simulink model "pump_original_discrete_filter"  (R2018a)
settings: Solver=VariableStepDiscrete  StartTime=0.0  StopTime=40  RelTol=1e-3
values from neighbouring files (symbols this model uses):
  Pl = 22    [pump_ori_perf.mat]
  Ts = 0.0001    [pump_ori_perf.mat]
undefined symbols (not defined in the file or in its folder): DiscIntNeverNeededParam
libraries: fl_lib x13, powerlib x7, powerlib_meascontrol x7, nesl_utility x6, sh_lib x4, simulink x3, dspstat3 x2
settings Model: SimulationMode=accelerator  Creator=siwak  LastModifiedBy=siwak
settings DataIOCC: ReturnWorkspaceOutputs=on
settings OptimizationCC: EfficientMapNaN2IntZero=off
settings DebuggingCC: ReadBeforeWriteMsg=DisableAll  WriteAfterWriteMsg=DisableAll  WriteAfterReadMsg=DisableAll  MultiTaskDSMMsg=none
settings HardwareCC: TargetBitPerPointer=64  TargetBitPerSizeT=64  TargetBitPerPtrDiffT=64  TargetLongLongMode=on  TargetIntDivRoundTo=Zero  TargetEndianess=LittleEndian  TargetWordSize=64  TargetHWDeviceType=MATLAB Host  ProdEqTarget=off
settings CodeAppCC: MaxIdLength=128
settings GRTTargetCC: TargetLangStandard=C89/C90 (ANSI)  CombineOutputUpdateFcns=off  GRTInterface=on

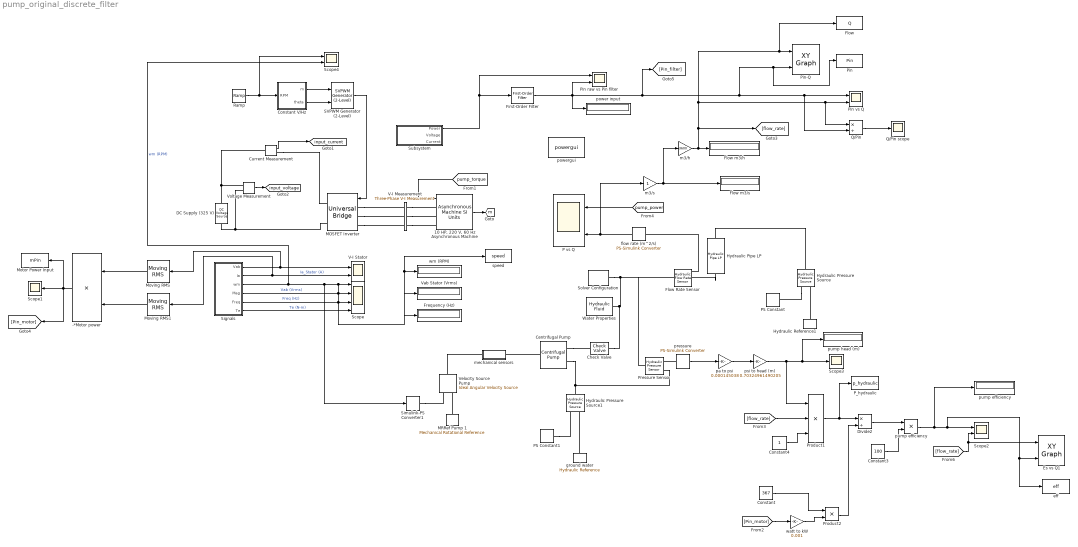
== system pump_original_discrete_filter ==
  " Flow Rate Sensor" : fl_lib/Hydraulic/Hydraulic Sensors/Hydraulic Flow Rate Sensor
      settings: SourceProductName=Simscape
  -*Motor power : Product
  "10 HP, 220 V, 60 Hz Asynchronous Machine" : powerlib/Machines/Asynchronous Machine SI Units  RotorType=Squirrel-cage  PresetModel=No  MechanicalLoad=Torque Tm  ShowDetailedParameters=on  ReferenceFrame=Stationary  Units=SI  MeasurementBus=off  NominalParameters=[ 10*746, 220, 60 ]  Stator="[ 0.435  2*2.0e-3 ]"  Rotor="[ 0.816  2.0e-3 ]"  Cage1=[ 0.022 0.226/377]  Cage2=[ 0.022 0.226/377]  Lm=69.31e-3  Mechanical="[ 0.089  0  2 ]"  PolePairs=2  InitialConditions=[1 90 0 0 0 0 0 0]  SimulateSaturation=off  Saturation=[0 0;0 0]  LoadFlowParameters=2000  TsPowergui=0  TsBlock=-1  IterativeModel=Trapezoidal non iterative  IterativeDiscreteModel=Trapezoidal non iterative  Pmec=0
  Centrifugal Pump : sh_lib/Pumps and Motors/Centrifugal Pump  mdl_type=2  c_1=326.8 Pa/(kg/m^3)  c_2=3.104e+4 Pa*s/kg  c_3=1.097e+7 Pa*s^2/(kg*m^3)  c_4=2.136e+5 Pa*s^2/(kg*m^3)  c_f=0.8  design_del=130 lpm  ref_velocity=1.70e+3 rpm  ref_density=940 kg/m^3  leak_resistance=1e+8 Pa/(m^3/s)  T_const=0.1 N*m  trq_press_coeff=1e-6 N*m/Pa  pump_del_1D="[0    0.0013    0.0041    0.0059    0.0069    0.0082] m^3/s"  press_diff_1D=[50.97 47.08 39.12 31.39 23.6 15.69] psi  pump_del_power_1D="[0    0.0013    0.0041    0.0059    0.0069    0.0082] m^3/s"  power_1D="[0    0.7800    2.1000    2.4000    2.1600    1.7000] HP"  pump_vel_2D=[ 3.2e+3 3.3e+3 3.4e+3 3.5e+3 ] rpm  pump_del_2D=[ 0 50 100 150 200 250 300 350 ] lpm  press_diff_2D=[ 8.3 8.8 9.3 9.9; 7.8 8.3 8.8 9.4; 7.2 7.6 8.2 8.7; 6.5 7 7.5 8; 5.6 6.1 6.6 7.1; 4.7 5.2 5.7 6.2; 3.4 4 4.4 4.9; 2.3 2.7 3.4 3.6 ] bar  pump_del_power_2D=[ 0 50 100 150 200 250 300 350 ] lpm  power_2D=[ 1.223e+3 1.341e+3 1.467e+3 1.6e+3; 1.414e+3 1.551e+3 1.696e+3 1.85e+3; 1.636e+3 1.794e+3 1.962e+3 2.14e+3; 1.941e+3 2.129e+3 2.326e+3 2.54e+3; 2.224e+3 2.439e+3 2.66e+3 2.91e+3; 2.453e+3 2.691e+3 2.947e+3 3.21e+3; 2.757e+3 3.024e+3 3.307e+3 3.608e+3; 2.945e+3 3.23e+3 3.533e+3 3.854e+3 ] W  omega_threshold=1e-9 rad/s  interp_method=1  extrap_method=1
      settings: SourceProductName=Simscape Fluids  SourceProductBaseCode=SH
  "Check Valve " : sh_lib/Valves/Directional Valves/Check Valve  area_max=50670.74790975 mm^2  pres_crack=0.01 psi  pres_max=0.1 psi  C_d=0.7  A_leak=1e-9 m^2  lam_spec=1  B_lam=0.999  Re_cr=12  dynamic=0  tau=0.1 s  area_init=1e-12 m^2
      settings: SourceProductName=Simscape Fluids  SourceProductBaseCode=SH
  Constant : Constant  Value=367
  Constant V/Hz : Subsystem
  Constant3 : Constant  Value=100
  Constant4 : Constant
  Current Measurement : powerlib/Measurements/Current Measurement  PhasorSimulation=off  OutputType=Magnitude  PSBequivalent=0
  DC Supply (325 V) : powerlib/Electrical Sources/DC Voltage Source  Amplitude=325  Measurements=None
  Divide2 : Product  Inputs=*/
  Es vs Q1 : simulink/Sinks/XY Graph  xmin=0  xmax=25  ymin=0  ymax=100  st=-1
  First-Order Filter : powerlib_meascontrol/Filters/First-Order Filter  FilterType=Lowpass  Tc=0.1551  Ts=Ts  Initialize=off  Vac_Init=[0, 0, 60]  Vdc_Init=0  PlotResponse=off  FreqRange="[0,  200,  1]"
      settings: SourceProductName=Simscape Power Systems
  Flow : ToWorkspace  VariableName=Q  SampleTime=-1
      settings: Save2DSignal=2-D array (concatenate along first dimension)
  Flow m3/h : Display
      settings: Decimation=2
  Flow m3/s : Display
      settings: Decimation=2
  Frequency (Hz) : Display
      settings: Format=bank  SampleTime=Ts*1000
  Hydraulic Pipe LP : sh_lib/Low-Pressure Blocks/Hydraulic Pipe LP  cs_type=1  d_in=10 in  area=1e-4 m^2  D_h=1.12e-2 m  s_factor=64  length=Pl m  length_ad=1 m  roughness=15e-6 m  Re_lam=2000  Re_turb=4000  elevation_A=-0.5 m  elevation_B=Pl-0.5 m  g=9.80665 m/s^2  wall_type=1  pr_r_coef=2e-12 m/Pa  time_const=0.01 s  k_sh=1.4  p0=0 Pa
      settings: SourceProductName=Simscape Fluids  SourceProductBaseCode=SH
  Hydraulic Pressure Source : fl_lib/Hydraulic/Hydraulic Sources/Hydraulic Pressure Source
      settings: SourceProductName=Simscape  SourceProductBaseCode=SS
  Hydraulic Pressure Source1 : fl_lib/Hydraulic/Hydraulic Sources/Hydraulic Pressure Source
      settings: SourceProductName=Simscape  SourceProductBaseCode=SS
  Hydraulic Reference1 : fl_lib/Hydraulic/Hydraulic Elements/Hydraulic Reference
      settings: SourceProductName=Simscape
  MOSFET Inverter : powerlib/Power Electronics/Universal Bridge  Arms=3  SnubberResistance=1e5  SnubberCapacitance=inf  Device=MOSFET / Diodes  Ron=0.2e-3  Lon=0  ForwardVoltages="[  0  0  ]"  ForwardVoltage=0  GTOparameters=[ 10e-6 , 20e-6 ]  IGBTparameters=[ 1e-6 , 2e-6 ]  Measurements=Device currents  Measurements_2=None  converterType=Rectifier
  MRRef Pump 1 : fl_lib/Mechanical/Rotational Elements/Mechanical Rotational Reference
  Motor Power Input : ToWorkspace  VariableName=mPin  SampleTime=-1
      settings: Save2DSignal=2-D array (concatenate along first dimension)
  Moving RMS : dspstat3/Moving RMS  Method=Sliding window  ForgettingFactorPort=off  SpecifyWindowLength=off  WindowLength=4  ForgettingFactor=0.9  SimulateUsing=Code generation
      settings: SourceProductName=DSP System Toolbox  SourceProductBaseCode=DS
  Moving RMS1 : dspstat3/Moving RMS  Method=Sliding window  ForgettingFactorPort=off  SpecifyWindowLength=off  WindowLength=4  ForgettingFactor=0.9  SimulateUsing=Code generation
      settings: SourceProductName=DSP System Toolbox  SourceProductBaseCode=DS
  P vs Q : Scope  NumInputPorts=2
  PS Constant : fl_lib/Physical Signals/Sources/PS Constant  constant=Pl/10
  PS Constant1 : fl_lib/Physical Signals/Sources/PS Constant  constant=0.2
  P_hydraulic : ToWorkspace  VariableName=p_hydraulic  SampleTime=-1
      settings: Save2DSignal=2-D array (concatenate along first dimension)
  Pin : ToWorkspace  VariableName=Pin  SampleTime=-1
      settings: Save2DSignal=2-D array (concatenate along first dimension)
  Pin raw vs Pin filter : Scope  NumInputPorts=2
  Pin vs Q : Scope  NumInputPorts=2
  Pin-Q : simulink/Sinks/XY Graph  xmin=0  xmax=25  ymin=0  ymax=2000  st=-1
  Pressure Sensor : fl_lib/Hydraulic/Hydraulic Sensors/Hydraulic Pressure Sensor
      settings: SourceProductName=Simscape
  Product1 : Product  Inputs=3
  Product2 : Product
  Q/Pin : Product  Inputs=*/  RndMeth=Nearest
  Q/Pin scope : Scope
  "Ramp " : simulink/Sources/Ramp  slope=30  start=10  InitialOutput=1000
  SVPWM Generator (2-Level) : powerlib_meascontrol/Pulse & Signal Generators/SVPWM Generator (2-Level)  InputType=Magnitude-Angle (rad)  SwitchingPattern=Pattern #1  Fc=1980  ParUref=[0.8 -30 50]  Ts=Ts
      settings: SourceProductName=Simscape Power Systems  SourceProductBaseCode=PS
  Scope : Scope  NumInputPorts=4
  Scope1 : Scope
  Scope2 : Scope  NumInputPorts=2
  Scope3 : Scope
  Scope4 : Scope  NumInputPorts=2
  Signals : Subsystem
  Simulink-PS Converter1 : nesl_utility/Simulink-PS Converter  PhysicalDomain=network_engine_domain  SubClassName=ps_input  LeftPortType=input  RightPortType=output  PseudoPeriodic=off  Frequencies=[]  NoiseDistribution=none  NoiseParameters=[]  Unit=rpm  AffineConversion=off  FilteringAndDerivatives=zero  SimscapeFilterOrder=1  InputFilterTimeConstant=.001  UdotUserProvided=0
  Solver Configuration : nesl_utility/Solver Configuration  PhysicalDomain=network_engine_domain  SubClassName=solver  LeftPortType=input  RightPortType=generic  Tones=[]  Harmonics=[]  SimulateNoise=off  Profile=off  UseLocalSampling=off  EnableSwitchedLinearOptims=on  FrequencyDomain=off  UseCCode=off  RelTol=0.001  AbsTol=1e-06  MinStep=1e-09  ToWorkspace=off  RevertToSquareIcSolve=off  NumHomotopyIterations=100  PhasorMode=off  PhasorModeNumHarmonics=1  DoDC=off  ResidualTolerance=1e-9  UseLocalSolver=on  LocalSolverChoice=NE_BACKWARD_EULER_ADVANCER  LocalSolverSampleTime=Ts  DoFixedCost=off  MaxNonlinIter=3  MaxModeIter=2  LinearAlgebra=Sparse  EquationFormulation=NE_TIME_EF  DelaysMemoryBudget=1024  AutomaticFiltering=on  FilteringTimeConstant=0.001
  Subsystem : Subsystem
  V-I Measurement : powerlib/Measurements/Three-Phase V-I Measurement  VoltageMeasurement=phase-to-phase  SetLabelV=on  LabelV=Vabc_Stator  Vpu=off  VpuLL=off  CurrentMeasurement=yes  SetLabelI=on  LabelI=Iabc_Stator  Ipu=off  Pbase=100e6  Vbase=500e3  OutputType=Magnitude  PhasorSimulation=off  PSBequivalent=0
  V-I Stator : Scope  NumInputPorts=2
  Vab Stator (Vrms) : Display
      settings: Format=bank  SampleTime=Ts*1000
  Velocity Source Pump : fl_lib/Mechanical/Mechanical Sources/Ideal Angular Velocity Source
  Voltage Measurement : powerlib/Measurements/Voltage Measurement  PhasorSimulation=off  OutputType=Magnitude  PSBequivalent=0
  Water Properties : sh_lib/Hydraulic Utilities/Hydraulic Fluid  DataSource=1  SelFluid=24  SysTemp=1  TrapAir=0.001  ViscDerFactor=1  range_error=2
      settings: SourceProductName=Simscape Fluids
  eff : ToWorkspace  VariableName=eff  SampleTime=-1
      settings: Save2DSignal=2-D array (concatenate along first dimension)
  flow rate (m^2/s) : nesl_utility/PS-Simulink Converter  PhysicalDomain=network_engine_domain  SubClassName=ps_output  LeftPortType=input  RightPortType=output  PseudoPeriodic=off  Frequencies=[]  Unit=m^3/s  AffineConversion=off
  ground water : fl_lib/Hydraulic/Hydraulic Elements/Hydraulic Reference
      settings: SourceProductName=Simscape
  m3/h : Gain  Gain=3600
  m3/s : Gain
  mechanical sensors : Subsystem
  pa to psi : Gain  Gain=0.000145038
  power input : Display
      settings: SampleTime=Ts*1000
  powergui : powerlib/powergui  Priority=2  SimulationMode=Discrete  SampleTime=Ts  frequency=60  Iterations=50  frequencyindice=60  Pbase=100e6  ErrMax=1e-4  UnitsV=kV  UnitsW=MW  buscounter=0  FunctionMessages=off  echomessages=off  EnableUseOfTLC=off  CurrentSourceSwitches=off  DisableSnubberDevices=off  DisableRonSwitches=off  DisableVfSwitches=off  DisplayEquations=off  SolverType=Tustin/Backward Euler (TBE)  Interpol=off  ExternalGateDelay=off  methode=off  Ts=100  x0status=blocks  SPID=off  SwTol=0  HookPort=off  RestoreLinks=warning  ResistiveCurrentMeasurement=off  Frange=[0:2:500]  Ylog=off  Xlog=on  ShowGrid=off  save=off  variable=ZData  structure=0  ZoomFFT=on  StartTime=0.0  cycles=1  DisplayStyle=1  fundamental=60  FreqAxis=off  MaxFrequency=1000  frequencyindicesteady=1  RmsSteady=1  display=off
  pressure : nesl_utility/PS-Simulink Converter  PhysicalDomain=network_engine_domain  SubClassName=ps_output  LeftPortType=input  RightPortType=output  PseudoPeriodic=off  Frequencies=[]  Unit=Pa  AffineConversion=off
  psi to head (m) : Gain  Gain=0.70324961490205
  pump efficiency : Product
  "pump efficiency " : Display
      settings: Decimation=2
  pump head (m) : Display
      settings: Decimation=2
  speed : ToWorkspace  VariableName=speed  SampleTime=-1
      settings: Save2DSignal=2-D array (concatenate along first dimension)
  watt to kW : Gain  Gain=0.001
  wm (RPM) : Display
      settings: SampleTime=Ts*1000
  tag scope: input_current=global, input_voltage=global, m=global
  wires:
  flow rate (m^2/s)/1 -> m3/s/1, P vs Q/2
  [pump_power] -> P vs Q/1
  m3/s/1 -> m3/h/1, Flow m3/s/1
  m3/h/1 -> Flow/1, Pin-Q/1, Q/Pin/1, Pin vs Q/2, [flow_rate], Flow m3/h/1
  "Ramp "/1 -> Scope4/1, Constant V/Hz/1(RPM)
  Signals/4(Mag) -> Scope/2, Vab Stator (Vrms)/1  "Vab (Vrms)"
  Signals/5(Freq) -> Scope/3, Frequency (Hz)/1  "Freq (Hz)"
  Signals/6(Te) -> Scope/4  "Te (N-m)"
  SVPWM Generator (2-Level)/1 -> MOSFET Inverter/1
  Signals/1(Vab) -> Moving RMS/1, V-I Stator/1
  Signals/2(Ia) -> Moving RMS1/1, V-I Stator/2  "Ia_Stator (A)"
  "10 HP, 220 V, 60 Hz Asynchronous Machine"/1 -> [m]
  Constant V/Hz/1(m) -> SVPWM Generator (2-Level)/1
  Constant V/Hz/2(theta) -> SVPWM Generator (2-Level)/2
  Signals/3(wm) -> Scope4/2, Simulink-PS Converter1/1, Scope/1, speed/1, wm (RPM)/1  "wm (RPM)"
  Current Measurement/1 -> [input_current]
  Voltage Measurement/1 -> [input_voltage]
  [pump_torque] -> "10 HP, 220 V, 60 Hz Asynchronous Machine"/1
  Constant4/1 -> Product1/3
  pressure/1 -> pa to psi/1
  Divide2/1 -> pump efficiency/1
  Constant3/1 -> pump efficiency/2
  Product2/1 -> Divide2/2
  Product1/1 -> P_hydraulic/1, Divide2/1
  [flow_rate] -> Es vs Q1/1, Scope2/2
  Constant/1 -> Product2/1
  pa to psi/1 -> psi to head (m)/1
  psi to head (m)/1 -> Product1/1, pump head (m)/1, Scope3/1
  [flow_rate] -> Product1/2
  pump efficiency/1 -> "pump efficiency "/1, eff/1, Es vs Q1/2, Scope2/1
  [Pin_motor] -> watt to kW/1
  watt to kW/1 -> Product2/2
  Subsystem/1(Power) -> First-Order Filter/1, Pin raw vs Pin filter/1
  Q/Pin/1 -> Q/Pin scope/1
  First-Order Filter/1 -> power input/1, Pin raw vs Pin filter/2, [Pin_filter], Pin/1, Pin-Q/2, Q/Pin/2, Pin vs Q/1
  Moving RMS1/1 -> -*Motor power/2
  Moving RMS/1 -> -*Motor power/1
  -*Motor power/1 -> [Pin_motor], Motor Power Input/1, Scope1/1
  connections:
  Simulink-PS Converter1/RConn1 -- Velocity Source Pump/RConn1
  MRRef Pump 1/LConn1 -- Velocity Source Pump/RConn2
  Hydraulic Pressure Source1/LConn1 -- Centrifugal Pump/RConn2 -- Pressure Sensor/RConn1
  " Flow Rate Sensor"/RConn1 -- flow rate (m^2/s)/LConn1
  Pressure Sensor/LConn1 -- " Flow Rate Sensor"/LConn1 -- Solver Configuration/RConn1 -- "Check Valve "/RConn1 -- Water Properties/RConn1
  Centrifugal Pump/RConn1 -- "Check Valve "/LConn1
  V-I Measurement/RConn3 -- "10 HP, 220 V, 60 Hz Asynchronous Machine"/LConn3
  MOSFET Inverter/LConn3 -- V-I Measurement/LConn3
  MOSFET Inverter/LConn1 -- V-I Measurement/LConn1
  MOSFET Inverter/LConn2 -- V-I Measurement/LConn2
  V-I Measurement/RConn2 -- "10 HP, 220 V, 60 Hz Asynchronous Machine"/LConn2
  V-I Measurement/RConn1 -- "10 HP, 220 V, 60 Hz Asynchronous Machine"/LConn1
  DC Supply (325 V)/LConn1 -- Voltage Measurement/LConn2 -- MOSFET Inverter/RConn2
  Current Measurement/RConn1 -- MOSFET Inverter/RConn1
  Current Measurement/LConn1 -- Voltage Measurement/LConn1 -- DC Supply (325 V)/RConn1
  Hydraulic Pipe LP/RConn1 -- Hydraulic Pressure Source/LConn1
  Hydraulic Pressure Source/RConn1 -- PS Constant/RConn1
  Hydraulic Pipe LP/LConn1 -- " Flow Rate Sensor"/RConn2
  Hydraulic Reference1/LConn1 -- Hydraulic Pressure Source/RConn2
  Centrifugal Pump/LConn1 -- mechanical sensors/RConn1
  mechanical sensors/LConn1 -- Velocity Source Pump/LConn1
  PS Constant1/RConn1 -- Hydraulic Pressure Source1/RConn1
  ground water/LConn1 -- Hydraulic Pressure Source1/RConn2
  pressure/LConn1 -- Pressure Sensor/RConn2

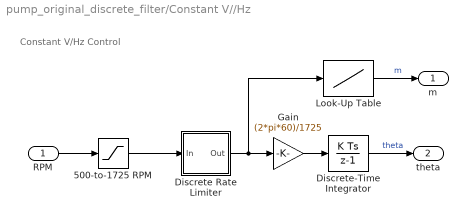
== system pump_original_discrete_filter/Constant V//Hz ==
  note: Constant V/Hz
      | Control
  RPM : Inport
  500-to-1725 RPM : Saturate  UpperLimit=1700  LowerLimit=500
  Discrete Rate Limiter : Subsystem  DialogController=POWERSYS.PowerSysDialog  mask(Discrete Rate Limiter){R=500, F=-500, Vinit=500, Ts=Ts}
      mask prompts: R "Rising slew rate:"; F "Falling slew rate:"; Vinit "Initial input:"; Ts "Sample time:"
      mask help: DISCRETE BLOCK : Limit rising and falling rates of signal
      mask init:
      | UpperLimit=R*Ts;
      | LowerLimit=F*Ts;
      | power_initmask();
      mask Display: disp('Discrete\nRate\nLimiter')
  Discrete-Time Integrator : DiscreteIntegrator  SampleTime=Ts  ICPrevOutput=DiscIntNeverNeededParam  ICPrevScaledInput=DiscIntNeverNeededParam
  Gain : Gain  Gain=(2*pi*60)/1725  SaturateOnIntegerOverflow=on  OutDataTypeStr=Inherit: Same as input  ParamDataTypeStr=Inherit: Same as input
  Look-Up Table : Lookup  InputValues=[500 1725 2500]  Table=[0.29 1 1]*0.957  SaturateOnIntegerOverflow=on
  m : Outport
  theta : Outport  Port=2
  wires:
  Gain/1 -> Discrete-Time Integrator/1
  Discrete Rate Limiter/1(Out) -> Gain/1, Look-Up Table/1
  Look-Up Table/1 -> m/1  "m"
  RPM/1 -> 500-to-1725 RPM/1
  Discrete-Time Integrator/1 -> theta/1  "theta"
  500-to-1725 RPM/1 -> Discrete Rate Limiter/1(In)

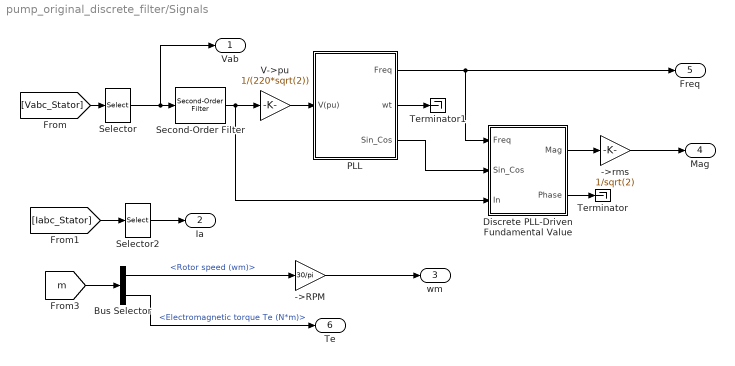
== system pump_original_discrete_filter/Signals ==
  ->RPM : Gain  Gain=30/pi  SaturateOnIntegerOverflow=on  OutDataTypeStr=Inherit: Same as input  ParamDataTypeStr=Inherit: Same as input
  ->rms : Gain  Gain=1/sqrt(2)  SaturateOnIntegerOverflow=on  OutDataTypeStr=Inherit: Same as input  ParamDataTypeStr=Inherit: Same as input
  Bus Selector : BusSelector  OutputSignals=Mechanical.Rotor speed (wm),Mechanical.Electromagnetic torque Te (N*m)
  Discrete PLL-Driven Fundamental Value : Subsystem  mask(Discrete PLL-Driven Fundamental Value){Finit=60, Par_Init=[220*sqrt(2) 0], Ts=Ts*20}
      mask prompts: Finit "Initial fundamental frequency (Hz):"; Par_Init "Initial input: [ Mag  Phase-relative-to-PLL(degrees) ]"; Ts "Sample time:"
      mask help:
      | This discrete block computes the fundamental value of the input signal (port In) over a running window of one cycle of a specified fundamental frequency (port Freq). Input port "Sin_Cos" (a two-dimension signal) provides the reference frame required for the computation..
      |  First and second outputs return respectively the magnitude and phase (in degrees relative to the PLL phase) of the fundamental.
      | For the first cycle of simulation, the outputs are held constant to the values specified by the parameter "Initial input".
      mask init:
      | Real_Init=Par_Init(1)*cos(pi/180*Par_Init(2));
      | Imag_Init=Par_Init(1)*sin(pi/180*Par_Init(2));
  PLL : Subsystem  mask(Discrete 1-phase PLL){Par_Init=[27.52 60], ParK=[120 2800], Ts=Ts*20}
      mask prompts: Par_Init "Initial input:[ Phase(degrees)   Frequency(Hz) ]"; ParK "Regulator gains [ Kp  Ki ]"; Ts "Sample time:"
      mask help:
      | This Phase Locked Loop (PLL) system can be used  to synchronize on a variable frequency sinusoidal signal.
      |
      | Input 1: Normalized input signal V(pu)
      |
      | Output 1:  Measured frequency (Hz) = w/(2pi)
      | Output 2:  Ramp w.t  varying between  0 and 2*pi, synchronized on the zero-crossing (rising) of  the input signal
      | Output 3: Vector [sin(wt) cos(wt)]
      mask init:
      | Kp=ParK(1);
      | Ki=ParK(2);
      | Phase_Init=Par_Init(1);
      | Finit=Par_Init(2);
  Second-Order Filter : powerlib_meascontrol/Filters/Second-Order Filter  FilterType=Lowpass  Fo=0.707  Zeta=0.707  Ts=Ts  Initialize=on  Vac_Init="[1 30  60]"  Vdc_Init=0  PlotResponse=off  FreqRange=[0, 500, 1]
      settings: SourceProductName=Simscape Power Systems  SourceProductBaseCode=PS
  Selector : Selector  InputPortWidth=3  IndexOptions=Index vector (dialog)  Indices=[1]  OutputSizes=1
  Selector2 : Selector  InputPortWidth=3  IndexOptions=Index vector (dialog)  Indices=[1]  OutputSizes=1
  Terminator : Terminator
  Terminator1 : Terminator
  V->pu : Gain  Gain=1/(220*sqrt(2))  SaturateOnIntegerOverflow=on  OutDataTypeStr=Inherit: Same as input  ParamDataTypeStr=Inherit: Same as input
  Vab : Outport
  Ia : Outport  Port=2
  wm : Outport  Port=3
  Mag : Outport  Port=4
  Freq : Outport  Port=5
  Te : Outport  Port=6
  wires:
  PLL/2(wt) -> Terminator1/1
  PLL/3(Sin_Cos) -> Discrete PLL-Driven Fundamental Value/2(Sin_Cos)
  V->pu/1 -> PLL/1(V(pu))
  Selector/1 -> Second-Order Filter/1, Vab/1
  Discrete PLL-Driven Fundamental Value/1(Mag) -> ->rms/1
  [Vabc_Stator] -> Selector/1
  [Iabc_Stator] -> Selector2/1
  ->RPM/1 -> wm/1
  ->rms/1 -> Mag/1
  Selector2/1 -> Ia/1
  Second-Order Filter/1 -> V->pu/1, Discrete PLL-Driven Fundamental Value/3(In)
  [m] -> Bus Selector/1
  Bus Selector/1 -> ->RPM/1  "<Rotor speed (wm)>"
  Bus Selector/2 -> Te/1  "<Electromagnetic torque Te (N*m)>"
  PLL/1(Freq) -> Discrete PLL-Driven Fundamental Value/1(Freq), Freq/1
  Discrete PLL-Driven Fundamental Value/2(Phase) -> Terminator/1

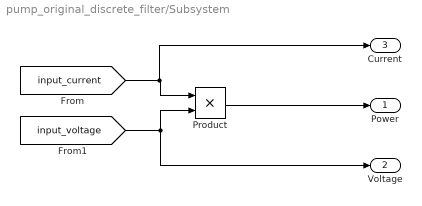
== system pump_original_discrete_filter/Subsystem ==
  Product : Product
  Power : Outport
  Voltage : Outport  Port=2
  Current : Outport  Port=3
  wires:
  Product/1 -> Power/1
  [input_current] -> Current/1, Product/1
  [input_voltage] -> Voltage/1, Product/2

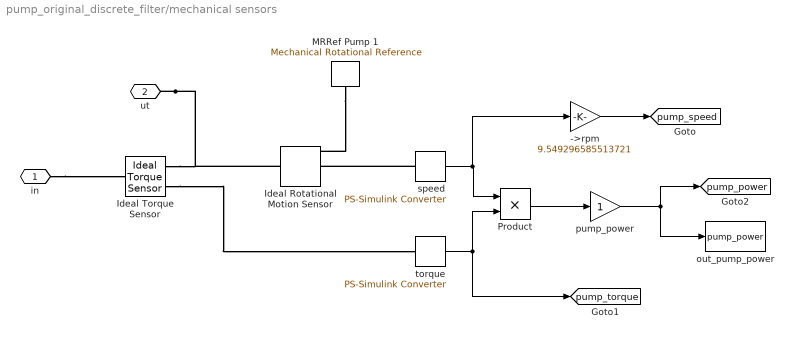
== system pump_original_discrete_filter/mechanical sensors ==
  ->rpm : Gain  Gain=9.549296585513721
  Ideal Rotational Motion Sensor : fl_lib/Mechanical/Mechanical Sensors/Ideal Rotational Motion Sensor  offset=0 rad
  Ideal Torque Sensor : fl_lib/Mechanical/Mechanical Sensors/Ideal Torque Sensor
  MRRef Pump 1 : fl_lib/Mechanical/Rotational Elements/Mechanical Rotational Reference
  Product : Product
  out_pump_power : ToWorkspace  VariableName=pump_power  SampleTime=-1
      settings: Save2DSignal=2-D array (concatenate along first dimension)
  pump_power : Gain
  speed : nesl_utility/PS-Simulink Converter  PhysicalDomain=network_engine_domain  SubClassName=ps_output  LeftPortType=input  RightPortType=output  PseudoPeriodic=off  Frequencies=[]  Unit=rad/s  AffineConversion=off
  torque : nesl_utility/PS-Simulink Converter  PhysicalDomain=network_engine_domain  SubClassName=ps_output  LeftPortType=input  RightPortType=output  PseudoPeriodic=off  Frequencies=[]  Unit=N*m  AffineConversion=off
  in : PMIOPort  Side=Left
  ut : PMIOPort  Port=2  Side=Right
  tag scope: pump_power=global, pump_speed=global, pump_torque=global
  wires:
  pump_power/1 -> out_pump_power/1, [pump_power]
  speed/1 -> ->rpm/1, Product/1
  Product/1 -> pump_power/1
  torque/1 -> Product/2, [pump_torque]
  ->rpm/1 -> [pump_speed]
  connections:
  ut/RConn1 -- Ideal Torque Sensor/RConn1 -- Ideal Rotational Motion Sensor/LConn1
  speed/LConn1 -- Ideal Rotational Motion Sensor/RConn2
  in/RConn1 -- Ideal Torque Sensor/LConn1
  MRRef Pump 1/LConn1 -- Ideal Rotational Motion Sensor/RConn1
  Ideal Torque Sensor/RConn2 -- torque/LConn1

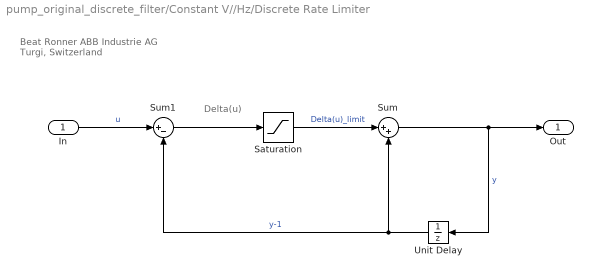
== system pump_original_discrete_filter/Constant V//Hz/Discrete Rate Limiter ==
  note: Beat Ronner
      | ABB Industrie AG
      | Turgi, Switzerland
  note: Delta(u)
  In : Inport
  Saturation : Saturate  UpperLimit=UpperLimit  LowerLimit=LowerLimit
  Sum : Sum  Inputs=|++  SaturateOnIntegerOverflow=on  InputSameDT=on  OutDataTypeStr=Inherit: Same as first input
  Sum1 : Sum  Inputs=|+-  SaturateOnIntegerOverflow=on  InputSameDT=on  OutDataTypeStr=Inherit: Same as first input
  Unit Delay : UnitDelay  InitialCondition=Vinit  SampleTime=Ts
  Out : Outport
  wires:
  Unit Delay/1 -> Sum/2, Sum1/2  "y-1"
  Sum/1 -> Unit Delay/1, Out/1  "y"
  Saturation/1 -> Sum/1  "Delta(u)_limit"
  Sum1/1 -> Saturation/1
  In/1 -> Sum1/1  "u"

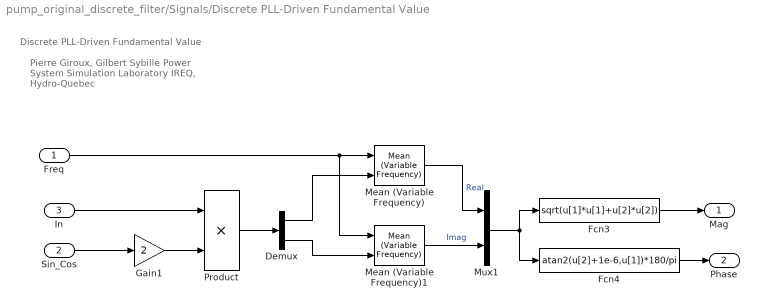
== system pump_original_discrete_filter/Signals/Discrete PLL-Driven Fundamental Value ==
  note: Discrete PLL-Driven Fundamental Value
  note: Pierre Giroux, Gilbert Sybille
      | Power System Simulation Laboratory
      | IREQ, Hydro-Quebec
  Freq : Inport
  Sin_Cos : Inport  Port=2
  In : Inport  Port=3
  Demux : Demux  Outputs=2
  Fcn3 : Fcn  Expr=sqrt(u[1]*u[1]+u[2]*u[2])
  Fcn4 : Fcn  Expr=atan2(u[2]+1e-6,u[1])*180/pi
  Gain1 : Gain  Gain=2  SaturateOnIntegerOverflow=on  OutDataTypeStr=Inherit: Same as input  ParamDataTypeStr=Inherit: Same as input
  Mean (Variable Frequency) : powerlib_meascontrol/Measurements/Mean (Variable Frequency)  Finit=Finit  Fmin=20  Vinit=Real_Init  Ts=Ts
      settings: SourceProductName=Simscape Power Systems  SourceProductBaseCode=PS
  Mean (Variable Frequency)1 : powerlib_meascontrol/Measurements/Mean (Variable Frequency)  Finit=Finit  Fmin=20  Vinit=Imag_Init  Ts=Ts
      settings: SourceProductName=Simscape Power Systems  SourceProductBaseCode=PS
  Mux1 : Mux  Inputs=2
  Product : Product  SaturateOnIntegerOverflow=on  InputSameDT=on  OutDataTypeStr=Inherit: Same as first input
  Mag : Outport
  Phase : Outport  Port=2
  wires:
  Mux1/1 -> Fcn3/1, Fcn4/1
  Fcn3/1 -> Mag/1
  Fcn4/1 -> Phase/1
  Mean (Variable Frequency)1/1 -> Mux1/2  "Imag"
  Mean (Variable Frequency)/1 -> Mux1/1  "Real"
  Demux/1 -> Mean (Variable Frequency)/2
  Gain1/1 -> Product/2
  Product/1 -> Demux/1
  Demux/2 -> Mean (Variable Frequency)1/2
  Freq/1 -> Mean (Variable Frequency)1/1, Mean (Variable Frequency)/1
  Sin_Cos/1 -> Gain1/1
  In/1 -> Product/1

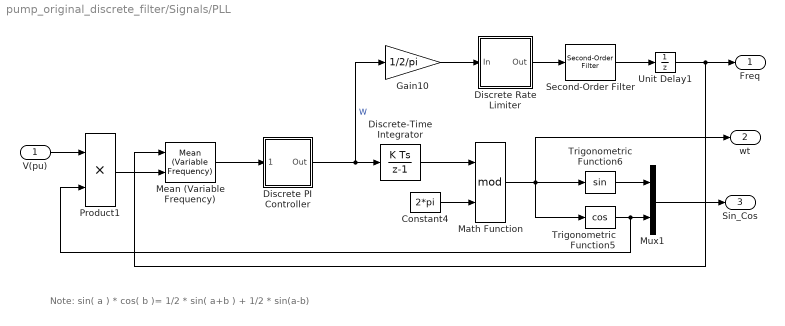
== system pump_original_discrete_filter/Signals/PLL ==
  note: Note: sin( a ) * cos( b )= 1/2 * sin( a+b ) + 1/2 * sin(a-b)
  V(pu) : Inport
  Constant4 : Constant  Value=2*pi
  Discrete PI Controller : Subsystem  DialogController=POWERSYS.PowerSysDialog  mask(Discrete PI Controller){Kp=Kp, Ki=Ki, Par_Limits=[4  0.25]*2*pi*Finit, Init=2*pi*Finit, Ts=Ts}
      mask prompts: Kp "Proportional gain (Kp):"; Ki "Integral gain (Ki):"; Par_Limits "Output limits: [ Upper   Lower ]"; Init "Output initial value:"; Ts "Sample time:"
      mask help: This block implements a discrete PI controller.
      mask init:
      | UpperLimit=Par_Limits(1);
      | LowerLimit=Par_Limits(2);
      | power_initmask();
      mask Display: disp('PI');
  Discrete Rate Limiter : Subsystem  DialogController=POWERSYS.PowerSysDialog  mask(Discrete Rate Limiter){R=30, F=-30, Vinit=Finit, Ts=Ts}
      mask prompts: R "Rising slew rate:"; F "Falling slew rate:"; Vinit "Initial input:"; Ts "Sample time:"
      mask help: DISCRETE BLOCK : Limit rising and falling rates of signal
      mask init:
      | UpperLimit=R*Ts;
      | LowerLimit=F*Ts;
      | power_initmask();
      mask Display: disp('Discrete\nRate\nLimiter')
  Discrete-Time Integrator : DiscreteIntegrator  InitialCondition=Phase_Init*pi/180  SampleTime=Ts  UpperSaturationLimit=0  LowerSaturationLimit=0  ICPrevOutput=DiscIntNeverNeededParam  ICPrevScaledInput=DiscIntNeverNeededParam
  Gain10 : Gain  Gain=1/2/pi  SaturateOnIntegerOverflow=on  OutDataTypeStr=Inherit: Same as input  ParamDataTypeStr=Inherit: Same as input
  Math Function : Math  Operator=mod  SaturateOnIntegerOverflow=on
  Mean (Variable Frequency) : powerlib_meascontrol/Measurements/Mean (Variable Frequency)  Finit=Finit  Fmin=10  Vinit=0  Ts=Ts
      settings: SourceProductName=Simscape Power Systems  SourceProductBaseCode=PS
  Mux1 : Mux  Inputs=2
  Product1 : Product  SaturateOnIntegerOverflow=on  InputSameDT=on  OutDataTypeStr=Inherit: Same as first input
  Second-Order Filter : powerlib_meascontrol/Filters/Second-Order Filter  FilterType=Lowpass  Fo=25  Zeta=0.707  Ts=Ts  Initialize=on  Vac_Init="[0 0  Finit]"  Vdc_Init=Finit  PlotResponse=off  FreqRange=[0, 500, 1]
      settings: SourceProductName=Simscape Power Systems  SourceProductBaseCode=PS
  Trigonometric Function5 : Trigonometry  Operator=cos
  Trigonometric Function6 : Trigonometry
  Unit Delay1 : UnitDelay  InitialCondition=Finit  SampleTime=Ts
  Freq : Outport
  wt : Outport  Port=2
  Sin_Cos : Outport  Port=3
  wires:
  Unit Delay1/1 -> Mean (Variable Frequency)/1, Freq/1
  Discrete PI Controller/1(Out) -> Gain10/1, Discrete-Time Integrator/1  "W"
  V(pu)/1 -> Product1/1
  Constant4/1 -> Math Function/2
  Discrete-Time Integrator/1 -> Math Function/1
  Product1/1 -> Mean (Variable Frequency)/2
  Mean (Variable Frequency)/1 -> Discrete PI Controller/1(Error)
  Mux1/1 -> Sin_Cos/1
  Math Function/1 -> Trigonometric Function6/1, Trigonometric Function5/1, wt/1
  Trigonometric Function6/1 -> Mux1/1
  Trigonometric Function5/1 -> Mux1/2, Product1/2
  Second-Order Filter/1 -> Unit Delay1/1
  Gain10/1 -> Discrete Rate Limiter/1(In)
  Discrete Rate Limiter/1(Out) -> Second-Order Filter/1

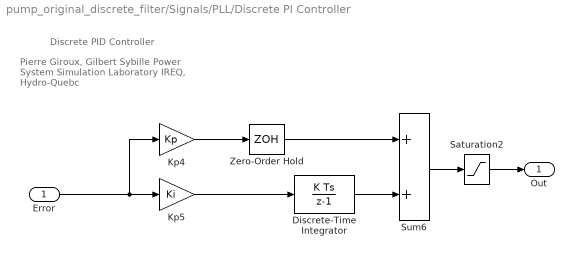
== system pump_original_discrete_filter/Signals/PLL/Discrete PI Controller ==
  note: Discrete PID Controller
  note: Pierre Giroux, Gilbert Sybille
      | Power System Simulation Laboratory
      | IREQ, Hydro-Quebc
  Error : Inport  SampleTime=Ts
  Discrete-Time Integrator : DiscreteIntegrator  InitialCondition=Init  SampleTime=Ts  LimitOutput=on  UpperSaturationLimit=UpperLimit  LowerSaturationLimit=LowerLimit  ICPrevOutput=DiscIntNeverNeededParam  ICPrevScaledInput=DiscIntNeverNeededParam
  Kp4 : Gain  Gain=Kp  SampleTime=Ts  SaturateOnIntegerOverflow=on  OutDataTypeStr=Inherit: Same as input  ParamDataTypeStr=Inherit: Same as input
  Kp5 : Gain  Gain=Ki  SampleTime=Ts  SaturateOnIntegerOverflow=on  OutDataTypeStr=Inherit: Same as input  ParamDataTypeStr=Inherit: Same as input
  Saturation2 : Saturate  UpperLimit=UpperLimit  LowerLimit=LowerLimit  SampleTime=Ts
  Sum6 : Sum  SampleTime=Ts  SaturateOnIntegerOverflow=on  InputSameDT=on  OutDataTypeStr=Inherit: Same as first input
  Zero-Order Hold : ZeroOrderHold  SampleTime=Ts
  Out : Outport  SampleTime=Ts  InitialOutput=0
  wires:
  Zero-Order Hold/1 -> Sum6/1
  Saturation2/1 -> Out/1
  Discrete-Time Integrator/1 -> Sum6/2
  Kp4/1 -> Zero-Order Hold/1
  Kp5/1 -> Discrete-Time Integrator/1
  Sum6/1 -> Saturation2/1
  Error/1 -> Kp5/1, Kp4/1

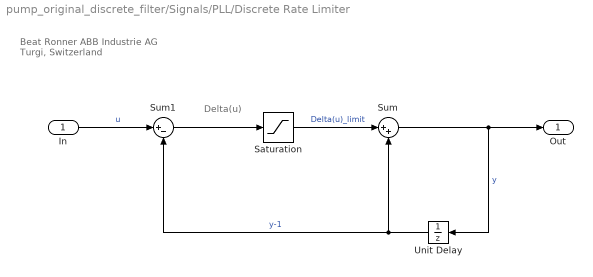
== system pump_original_discrete_filter/Signals/PLL/Discrete Rate Limiter ==
  note: Beat Ronner
      | ABB Industrie AG
      | Turgi, Switzerland
  note: Delta(u)
  In : Inport
  Saturation : Saturate  UpperLimit=UpperLimit  LowerLimit=LowerLimit
  Sum : Sum  Inputs=|++  SaturateOnIntegerOverflow=on  InputSameDT=on  OutDataTypeStr=Inherit: Same as first input
  Sum1 : Sum  Inputs=|+-  SaturateOnIntegerOverflow=on  InputSameDT=on  OutDataTypeStr=Inherit: Same as first input
  Unit Delay : UnitDelay  InitialCondition=Vinit  SampleTime=Ts
  Out : Outport
  wires:
  Unit Delay/1 -> Sum/2, Sum1/2  "y-1"
  Sum/1 -> Unit Delay/1, Out/1  "y"
  Saturation/1 -> Sum/1  "Delta(u)_limit"
  Sum1/1 -> Saturation/1
  In/1 -> Sum1/1  "u"
